simulink model "Test_Counter_2bit"  (R2016a)
settings: Solver=VariableStepAuto  StartTime=0.0  StopTime=100.0  RelTol=1e-3
libraries: commutil2 x1, simulink_extras x1, Clock_Lib x1
settings Model: Creator=Jozko Mrkvicka  LastModifiedBy=Jozko Mrkvicka

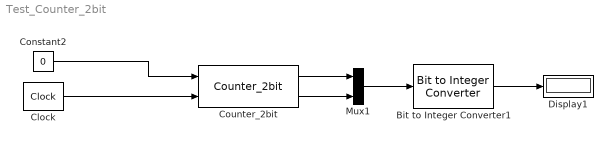
== system Test_Counter_2bit ==
  Bit to Integer Converter1 : commutil2/Bit to Integer Converter  nbits=2  bitOrder=MSB first  signedOutputValues=Unsigned  outDtype=uint8  outDtypeSigned=Inherit via internal rule
  Clock : simulink_extras/Flip Flops/Clock  period=2
  Constant2 : Constant  Value=0
  Counter_2bit : Clock_Lib/Counter_2bit
  Display1 : Display
  Mux1 : Mux  Inputs=2
  wires:
  Clock/1 -> Counter_2bit/2
  Constant2/1 -> Counter_2bit/1
  Counter_2bit/1 -> Mux1/1
  Counter_2bit/2 -> Mux1/2
  Mux1/1 -> Bit to Integer Converter1/1
  Bit to Integer Converter1/1 -> Display1/1
